simulink model "MPCS_3D_Formulation"  (R2016a)
settings: Solver=FixedStepAuto  StartTime=0.0  StopTime=30  FixedStep=Ts  RelTol=1e-3
InitFcn:
  | Ts = 0.005;
libraries: slrtlib x5
settings Model: SimulationMode=external  Creator=SLRT  LastModifiedBy=SLRT
settings SolverCC: EnableConcurrentExecution=on
settings DataIOCC: SaveFormat=StructureWithTime
settings OptimizationCC: BlockReduction=off  OptimizeBlockIOStorage=off  BufferReuse=off  GlobalBufferReuse=off  ExpressionFolding=off  LocalBlockOutputs=off
settings HardwareCC: ProdBitPerPointer=32  ProdLargestAtomicFloat=None  ProdWordSize=32  ProdLongLongMode=on  ProdHWDeviceType=Generic->32-bit x86 compatible
settings RTWCC: SystemTargetFile=slrt.tlc  TemplateMakefile=slrt_default_tmf  Description=Simulink Real-Time  RTWCompilerOptimization=on
settings RTWCC: CustomInclude=|
  | C:\Users\SLRT\Desktop\Swift\include
  | C:\Users\SLRT\Desktop\Swift\ldl\include
settings RTWCC: CustomSource=|
  | C:\Users\SLRT\Desktop\Swift\ldl\src\ldl.c
  | C:\Users\SLRT\Desktop\Swift\src\Auxilary.c
  | C:\Users\SLRT\Desktop\Swift\src\Prime.c
  | C:\Users\SLRT\Desktop\Swift\src\timer.c

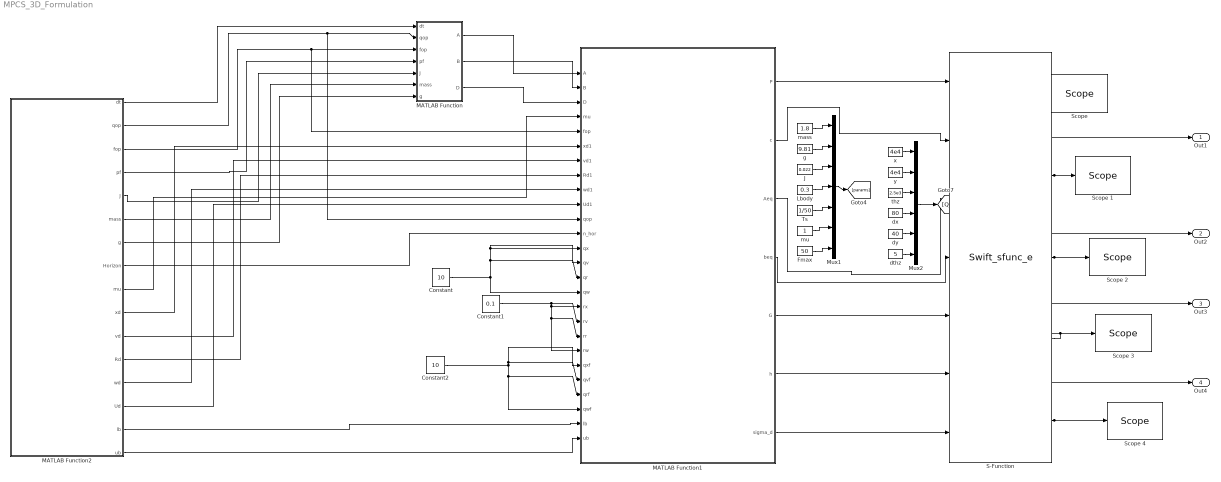
== system MPCS_3D_Formulation ==
  Constant : Constant  Value=10
  Constant1 : Constant  Value=0.1
  Constant2 : Constant  Value=10
  Fmax : Constant  Value=50  SampleTime=Ts
  J : Constant  Value=0.022  SampleTime=Ts
  Lbody : Constant  Value=0.3  SampleTime=Ts
  MATLAB Function : MATLAB Function  TreatAsAtomicUnit=on
  MATLAB Function1 : MATLAB Function  TreatAsAtomicUnit=on
  MATLAB Function2 : MATLAB Function  TreatAsAtomicUnit=on
  Mux1 : Mux  Inputs=7
  Mux2 : Mux  Inputs=6
  S-Function : S-Function  FunctionName=Swift_sfunc_e  SFunctionDeploymentMode=off  EnableBusSupport=off
  "Scope " : slrtlib/Displays and Logging/Scope   scopeno=1  scopetype=Target  autostart=on  viewmode=Numerical  formatstr='%15.6f'  grid=on  ylimits=[0,0]  nosamples=3  noprepostsamples=0  interleave=1  triggermode=FreeRun  triggersignal=1  trigsignalfromport=off  triggerlevel=0.0  triggerslope=Either  triggerscope=1  triggersample=0  filename=data.dat  mode=Lazy  writesize=512  autorestart=off  dynamicfilemode=off  maxwritefilesize=512*1024^2
  Scope 1 : slrtlib/Displays and Logging/Scope   scopeno=2  scopetype=Target  autostart=on  viewmode=Numerical  formatstr='%15.6f'  grid=on  ylimits=[0,0]  nosamples=3  noprepostsamples=0  interleave=1  triggermode=FreeRun  triggersignal=1  trigsignalfromport=off  triggerlevel=0.0  triggerslope=Either  triggerscope=1  triggersample=0  filename=data.dat  mode=Lazy  writesize=512  autorestart=off  dynamicfilemode=off  maxwritefilesize=512*1024^2
  Scope 2 : slrtlib/Displays and Logging/Scope   scopeno=3  scopetype=Target  autostart=on  viewmode=Numerical  formatstr='%15.6f'  grid=on  ylimits=[0,0]  nosamples=3  noprepostsamples=0  interleave=1  triggermode=FreeRun  triggersignal=1  trigsignalfromport=off  triggerlevel=0.0  triggerslope=Either  triggerscope=1  triggersample=0  filename=data.dat  mode=Lazy  writesize=512  autorestart=off  dynamicfilemode=off  maxwritefilesize=512*1024^2
  Scope 3 : slrtlib/Displays and Logging/Scope   scopeno=4  scopetype=Target  autostart=on  viewmode=Numerical  formatstr='%15.6f'  grid=on  ylimits=[0,0]  nosamples=3  noprepostsamples=0  interleave=1  triggermode=FreeRun  triggersignal=1  trigsignalfromport=off  triggerlevel=0.0  triggerslope=Either  triggerscope=1  triggersample=0  filename=data.dat  mode=Lazy  writesize=512  autorestart=off  dynamicfilemode=off  maxwritefilesize=512*1024^2
  Scope 4 : slrtlib/Displays and Logging/Scope   scopeno=5  scopetype=Target  autostart=on  viewmode=Numerical  formatstr='%15.6f'  grid=on  ylimits=[0,0]  nosamples=3  noprepostsamples=0  interleave=1  triggermode=FreeRun  triggersignal=1  trigsignalfromport=off  triggerlevel=0.0  triggerslope=Either  triggerscope=1  triggersample=0  filename=data.dat  mode=Lazy  writesize=512  autorestart=off  dynamicfilemode=off  maxwritefilesize=512*1024^2
  Ts : Constant  Value=1/50  SampleTime=Ts
  dthz : Constant  Value=5  SampleTime=Ts
  dx : Constant  Value=80  SampleTime=Ts
  dy : Constant  Value=40  SampleTime=Ts
  g : Constant  Value=9.81  SampleTime=Ts
  mass : Constant  Value=1.8  SampleTime=Ts
  mu : Constant  SampleTime=Ts
  thz : Constant  Value=2.5e3  SampleTime=Ts
  x : Constant  Value=4e4  SampleTime=Ts
  y : Constant  Value=4e4  SampleTime=Ts
  Out1 : Outport
  Out2 : Outport  Port=2
  Out3 : Outport  Port=3
  Out4 : Outport  Port=4
  wires:
  MATLAB Function/1(A) -> MATLAB Function1/1(A)
  MATLAB Function/2(B) -> MATLAB Function1/2(B)
  MATLAB Function/3(D) -> MATLAB Function1/3(D)
  MATLAB Function2/1(dt) -> MATLAB Function/1(dt)
  MATLAB Function2/2(qop) -> MATLAB Function1/11(qop), MATLAB Function/2(qop)
  MATLAB Function2/3(fop) -> MATLAB Function1/5(fop), MATLAB Function/3(fop)
  MATLAB Function2/4(pf) -> MATLAB Function/4(pf)
  MATLAB Function2/5(J) -> MATLAB Function/5(J)
  MATLAB Function2/6(mass) -> MATLAB Function/6(mass)
  MATLAB Function2/7(g) -> MATLAB Function/7(g)
  MATLAB Function2/9(mu) -> MATLAB Function1/4(mu)
  MATLAB Function2/8(Horizon) -> MATLAB Function1/12(n_hor)
  MATLAB Function2/15(lb) -> MATLAB Function1/25(lb)
  MATLAB Function2/16(ub) -> MATLAB Function1/26(ub)
  MATLAB Function2/14(Ud) -> MATLAB Function1/10(Ud1)
  MATLAB Function2/13(wd) -> MATLAB Function1/9(wd1)
  MATLAB Function2/12(Rd) -> MATLAB Function1/8(Rd1)
  MATLAB Function2/11(vd) -> MATLAB Function1/7(vd1)
  MATLAB Function2/10(xd) -> MATLAB Function1/6(xd1)
  Constant/1 -> MATLAB Function1/14(qv), MATLAB Function1/13(qx), MATLAB Function1/15(qr), MATLAB Function1/16(qw)
  Constant1/1 -> MATLAB Function1/20(rw), MATLAB Function1/19(rr), MATLAB Function1/17(rx), MATLAB Function1/18(rv)
  Constant2/1 -> MATLAB Function1/21(qxf), MATLAB Function1/22(qvf), MATLAB Function1/24(qwf), MATLAB Function1/23(qrf)
  MATLAB Function1/1(P) -> S-Function/1
  MATLAB Function1/2(c) -> S-Function/2
  MATLAB Function1/3(Aeq) -> S-Function/3
  MATLAB Function1/4(beq) -> S-Function/4
  MATLAB Function1/5(G) -> S-Function/5
  MATLAB Function1/6(h) -> S-Function/6
  MATLAB Function1/7(sigma_d) -> S-Function/7
  S-Function/3 -> Out2/1, Scope 2/1
  S-Function/2 -> Out1/1, Scope 1/1
  S-Function/5 -> Out4/1, Scope 4/1
  mass/1 -> Mux1/1
  g/1 -> Mux1/2
  J/1 -> Mux1/3
  Lbody/1 -> Mux1/4
  Ts/1 -> Mux1/5
  Mux1/1 -> [params]
  Mux2/1 -> [Q_co]
  mu/1 -> Mux1/6
  Fmax/1 -> Mux1/7
  x/1 -> Mux2/1
  y/1 -> Mux2/2
  thz/1 -> Mux2/3
  dx/1 -> Mux2/4
  dy/1 -> Mux2/5
  dthz/1 -> Mux2/6
  S-Function/1 -> "Scope "/1
  S-Function/4 -> Out3/1, Scope 3/1

== matlab function MPCS_3D_Formulation/MATLAB Function1 ==
  data: A input; B input; D input; mu input; fop input; xd1 input; vd1 input; Rd1 input; wd1 input; Ud1 input; qop input; n_hor input; qx input; qv input; qr input; qw input; rx input; rv input; rr input; rw input; qxf input; qvf input; qrf input; qwf input; lb input; ub input; P output; c output; Aeq output; beq output; G output; h output; sigma_d output
function [P,c,Aeq,beq,G,h,sigma_d] = Custom_QP_Form(A,B,D,mu,fop,xd1,vd1,Rd1,wd1,Ud1,qop,n_hor,qx,qv,qr,qw,rx,rv,rr,rw,qxf,qvf,qrf,qwf,lb,ub)
%n_hor
%xd = [xd1 .... xd_n_hor];
%vd = [vd1 .... vd_n_hor];
%wd = [wd1 .... wd_n_hor];
%Rd(:,:,1) = Rd1, Rd(:,:,n_hor) = Rd_n_hor
% if desired values are only one values, then assumes constant desired
% values
%Ud = [Ud1 .... Ud_n_hor];
%Model: x_(k+1)=A*x_k+B*u_k+D
%mu: friction cone, pyramid 
%qop: operating point q
%fop: operating point f
%ub = [uu1... uun_hor];
%lb = [ll1... lln_hor];
n_hor =7;
if size(xd1,2)==1
    xd = repmat(xd1,[1,n_hor]);
end
if size(vd1,2)==1
    vd = repmat(vd1,[1,n_hor]);
end
if size(wd1,2)==1
    wd = repmat(wd1,[1,n_hor]);
end
if size(Rd1,3)==1
    Rd = repmat(Rd1,[1,1,n_hor]);
end
if size(Ud1,2)==1
    Ud = repmat(Ud1,[1,n_hor]);
end
if size(ub,2)==1
    ub = repmat(ub,[1,n_hor]);
end
if size(lb,2)==1
    lb = repmat(lb,[1,n_hor]);
end
Some = [1,0,0,0,0,0,0,0,0;0,0,0,1,0,0,0,0,0;0,0,0,0,0,0,1,0,0;0,1,0,0,0,0,0,0,0;0,0,0,0,1,0,0,0,0;0,0,0,0,0,0,0,1,0;0,0,1,0,0,0,0,0,0;0,0,0,0,0,1,0,0,0;0,0,0,0,0,0,0,0,1];
L = zeros(9,9,n_hor);
for ii=1:n_hor
    L(:,:,ii) = 0.5*(kron(eye(3),Rd(:,:,ii)')-(kron(Rd(:,:,ii)',eye(3))*Some));
end

Vmap = [0 0 0 0 0 1 0 0 0;0 0 -1 0 0 0 0 0 0;0 1 0 0 0 0 0 0 0];
F_Rdwd = zeros(3,9,n_hor);
for ii=1:n_hor
    F_Rdwd(:,:,ii) = calculate_F(Rd(:,:,ii)*wd(:,ii));
end
n_inputs = 12;
n_states = 18;

Qx = qx*eye(3);
Qv = qv*eye(3);
Qr = qr*eye(3);
Qw = qw*eye(3);
Rx = rx*eye(3);
Rv = rv*eye(3);
Rr = rr*eye(3);
Rw = rw*eye(3);
Qxf = qxf*eye(3);
Qvf = qvf*eye(3);
Qrf = qrf*eye(3);
Qwf = qwf*eye(3);

Phi_w = F_Rdwd;
Phi_R = zeros(3,9,n_hor);
for ii=1:n_hor
    Phi_R(:,:,ii) = Vmap*L(:,:,ii);
end
Q = zeros(n_states,n_states,n_hor);
R = zeros(n_inputs,n_inputs,n_hor);
g1q = zeros(n_states,n_hor);
g1r = zeros(n_inputs,n_hor);
R1 = blkdiag(Rx,Rv,Rr,Rw);
for ii=1:n_hor
    if ii==n_hor
        Q(:,:,ii) = blkdiag(Qxf,Qvf,[Phi_R(:,:,ii)'*Qrf*Phi_R(:,:,ii)+Phi_w(:,:,ii)'*Qwf*Phi_w(:,:,ii) -Phi_w(:,:,ii)'*Qwf;-Qwf*Phi_w(:,:,ii) Qwf]);
    else
        Q(:,:,ii) = blkdiag(Qx,Qv,[Phi_R(:,:,ii)'*Qr*Phi_R(:,:,ii)+Phi_w(:,:,ii)'*Qw*Phi_w(:,:,ii) -Phi_w(:,:,ii)'*Qw;-Qw*Phi_w(:,:,ii) Qw]);
    end
    R(:,:,ii) = R1;
end
for ii=1:n_hor
    g1q(:,ii) = [-2*Qx'*xd(:,ii);-2*Qv'*vd(:,ii);zeros(9,1);zeros(3,1)];
    g1r(:,ii) = [2*R1'*(fop-Ud(:,ii))];
end
H = zeros([(n_states+n_inputs)*n_hor,(n_states+n_inputs)*n_hor]);
g = zeros([(n_states+n_inputs)*n_hor,1]);
for ii=1:n_hor
    idx_R = [1:n_inputs]+(ii-1)*(n_states+n_inputs);
    idx_Q = (ii-1)*(n_states+n_inputs) + n_inputs+ [1:n_states];
    H(idx_R,idx_R) = R(:,:,ii);
    H(idx_Q,idx_Q) = Q(:,:,ii);
    g(idx_R) = g1r(:,ii);
    g(idx_Q) = g1q(:,ii);
end
% H = blkdiag(R1,Q1,R1,Q1,R1,Q1,R1,Q1,R1,Q1,R1,Q1,R1,Q1);
% g = [g1r;g1q;g1r;g1q;g1r;g1q;g1r;g1q;g1r;g1q;g1r;g1q;g1r;g1q];
Fu = zeros(24,12);
Fu_x = [1 0 -mu;-1 0 -mu];
Fu_y = [0 1 -mu;0 -1 -mu];

Fu(1:4,1:3) = [Fu_x;Fu_y];
Fu(5:8,4:6) = [Fu_x;Fu_y];
Fu(9:12,7:9) = [Fu_x;Fu_y];
Fu(13:16,10:12) = [Fu_x;Fu_y];
Fu(17:18,1:3) = [0 0 1; 0 0 -1];
Fu(19:20,4:6) = [0 0 1; 0 0 -1];
Fu(21:22,7:9) = [0 0 1; 0 0 -1];
Fu(23:24,10:12) = [0 0 1; 0 0 -1];


F = zeros((16+8)*n_hor,30*n_hor);
for ii=1:n_hor
    F(24*(ii-1)+[1:24],(n_states+n_inputs)*(ii-1)+[1:n_inputs]) = Fu;
end

h1 = zeros(16,1);
for ii=1:4
    h1(4*(ii-1)+[1:4]) = [mu*fop(3+3*(ii-1))-fop(1+3*(ii-1));mu*fop(3+3*(ii-1))+fop(1+3*(ii-1));mu*fop(3+3*(ii-1))-fop(2+3*(ii-1));mu*fop(3+3*(ii-1))+fop(2+3*(ii-1))];
end
h = zeros(24*n_hor,1);
for ii=1:n_hor
    h(24*(ii-1)+[1:16]) = h1;       
    h(24*(ii-1)+[17:18]) = [ub(1,ii)-fop(3)+Ud(3,ii);-lb(1,ii)+fop(3)-Ud(3,ii)];
    h(24*(ii-1)+[19:20]) = [ub(2,ii)-fop(6)+Ud(6,ii);-lb(2,ii)+fop(6)-Ud(6,ii)];
    h(24*(ii-1)+[21:22]) = [ub(3,ii)-fop(9)+Ud(9,ii);-lb(3,ii)+fop(9)-Ud(9,ii)];
    h(24*(ii-1)+[23:24]) = [ub(4,ii)-fop(12)+Ud(12,ii);-lb(4,ii)+fop(12)-Ud(12,ii)];

end
%h = [h1;h1;h1;h1;h1;h1;h1];
C = zeros(n_states*n_hor,(n_states+n_inputs)*n_hor);
C(1:n_states,1:n_inputs) = -B;
C(1:n_states,n_inputs+[1:n_states]) = eye(n_states);
for ii=1:n_hor-1
    C(ii*n_states+[1:n_states],(ii-1)*(n_inputs+n_states)+n_inputs+[1:n_states]) = -A;
    C(ii*n_states+[1:n_states],(ii-1)*(n_inputs+n_states)+(n_inputs+n_states)+[1:n_inputs]) = -B;
    C(ii*n_states+[1:n_states],(ii-1)*(n_inputs+n_states)+(2*n_inputs+n_states)+[1:n_states]) = eye(n_states);
end
b = zeros(n_states*n_hor,1);
for ii=1:n_hor
    if ii==1
        b((ii-1)*n_states +[1:n_states]) = A*qop+D;
    else
        b((ii-1)*n_states +[1:n_states]) = D;
    end
end

eye_ = zeros(size(H,1),1);
idx_x= repmat([n_inputs+[7:n_states]]',[1 n_hor]) +repmat((0:(n_inputs+n_states):(n_hor-1)*(n_inputs+n_states)),[12,1]);
eye_(reshape(idx_x,[size(idx_x,1)*size(idx_x,2),1])) = 1e-5;

%[z,nu,fval,iter,Pr_feas,Dual_feas,no_Ineq_vio]= customQP_PredCorr(2*(H+diag(eye_)),g,F,h,C,b,n_hor,0);

% [z,nu,fval,iter,Pr_feas,Dual_feas,no_Ineq_vio]= customQP_PredCorr_full(2*(H+diag(eye_)),g,F,h,C,b,0);
% P = 2*(H + diag(eye_))(:):
% size(P)
% c = g;
% G = F(:);
% A = C(:);
% size(C)
% size(A)
M = 2*(H + diag(eye_));
P = M(:);
G = F(:);
c = g;
Aeq = C(:);
beq = b;
sigma_d = 0;

== matlab function MPCS_3D_Formulation/MATLAB Function ==
  data: dt input; A output; qop input; fop input; pf input; J input; mass input; g input; B output; D output
function [A,B,D] = complete(dt,qop,fop,pf,J,mass,g)
xop = qop(1:3,1);
vop = qop(4:6,1);
Rop = reshape(qop(7:15,1),[3,3]);
wop = qop(16:18,1);

    [c1,c2,c3] = coeffR(Rop,wop,dt);
    [a1,a2] = coeffx(dt);
    [b1 b2 b3] = coeffv(dt,mass,g,fop);
    [d1 d2 d3 d4 d5] = coeffw(Rop,wop,pf,dt,J,fop,xop);
    
    
    A = [a1,a2,zeros(3,12);zeros(3,3),b1,zeros(3,12);zeros(9,6),c1,c2;d1,zeros(3,3),d2,d3];

    B = [zeros(3,12);b2;zeros(9,12);d4];

    D = [zeros(3,1);b3;c3;d5];
    


end

== matlab function MPCS_3D_Formulation/MATLAB Function2 ==
  data: dt output; qop output; fop output; pf output; J output; mass output; g output; Horizon output; mu output; xd output; vd output; Rd output; wd output; Ud output; lb output; ub output
function [dt,qop,fop,pf,J,mass,g,Horizon,mu,xd,vd,Rd,wd,Ud,lb,ub] = fcn_settings

dt = 0.005;
[g,mass,J,pf] = my_params();

Horizon = 7;
mu = 1;
n_states = 18;
n_inputs = 12;
Rop = expm(my_hat(randn(3,1)));
% Rop = [-0.9179 0.3621 
xop = rand(3,1);
vop = rand(3,1);
wop = 0.1*rand(3,1);
Ud = repmat([0;0;5],[4,1]);
fop = Ud+1*rand(12,1);
xd = rand(3,1);
vd = rand(3,1);
Rd = rand(3,3);
wd = rand(3,1);


lb = -1*ones(4,Horizon);
ub = 1*ones(4,Horizon);

qop = [xop;vop;reshape(Rop,[9,1]);wop];
